simulink model "RLC"  (R2024b)
settings: Solver=VariableStepAuto  StartTime=0.0  StopTime=5.0  RelTol=1e-3
settings Model: Creator=viete  LastModifiedBy=viete

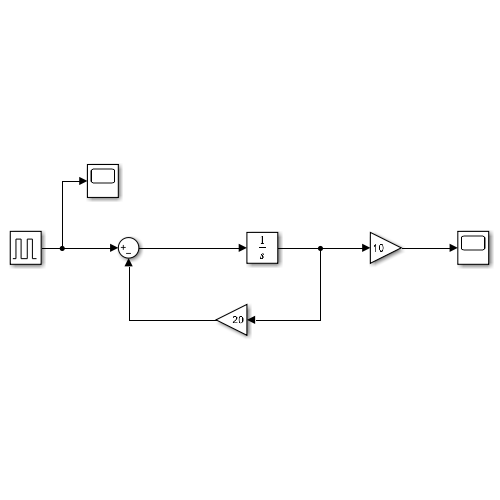
[thumbnail: Simulink's stored preview of the top-level diagram]
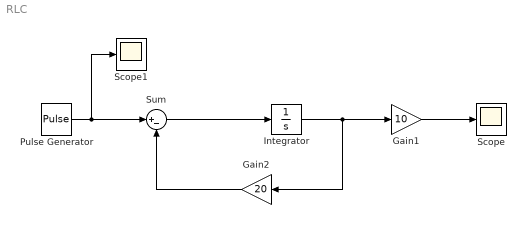
== system RLC ==
  Gain1 : Gain  Gain=10
  Gain2 : Gain  Gain=20
  Integrator : Integrator
  Pulse Generator : DiscretePulseGenerator  PulseType=Time based  Period=1  PulseWidth=50
  Scope : Scope
  Scope1 : Scope
  Sum : Sum  Inputs=|+-
  wires:
  Sum/1 -> Integrator/1
  Integrator/1 -> Gain2/1, Gain1/1
  Gain2/1 -> Sum/2
  Pulse Generator/1 -> Scope1/1, Sum/1
  Gain1/1 -> Scope/1
